simulink model "EOM_planar_vehicle"  (R2025b)
settings: Solver=VariableStepAuto  StartTime=0.0  StopTime=t_final  MaxStep=deltaTMax  RelTol=1e-3
undefined symbols (not defined in the file or in its folder): ENVIRONMENT, GEOMETRY, PROPULSION, SIMULATION
settings Model: Creator=nuris  LastModifiedBy=nuris
settings DataIOCC: ReturnWorkspaceOutputs=off

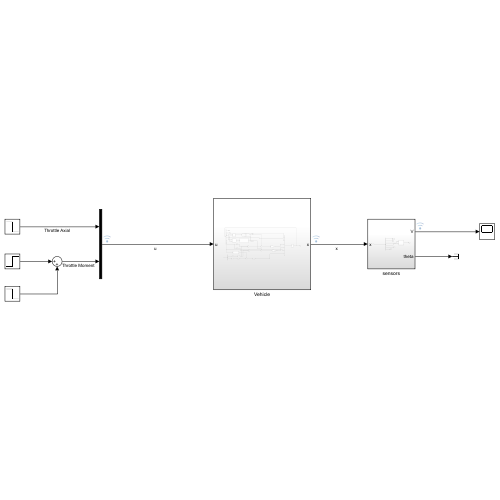
[thumbnail: Simulink's stored preview of the top-level diagram]
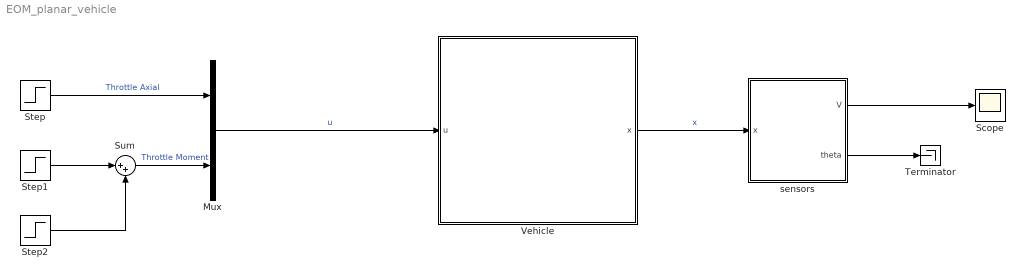
== system EOM_planar_vehicle ==
  Mux : Mux  Inputs=2
  Scope : Scope
      settings: ActiveDisplayYMinimum=-1.0187214318443125  ActiveDisplayYMaximum=20.5772184986616
  Step : Step  Time=90  Before=1  After=0  SampleTime=0
  Step1 : Step  Time=10  SampleTime=0
  Step2 : Step  Time=30  After=-1  SampleTime=0
  Sum : Sum  Inputs=|++
  Terminator : Terminator
  Vehicle : Subsystem
  sensors : Subsystem
  wires:
  Step2/1 -> Sum/2
  Step1/1 -> Sum/1
  Sum/1 -> Mux/2  "Throttle Moment"
  Step/1 -> Mux/1  "Throttle Axial"
  Mux/1 -> Vehicle/1(u)  "u"
  Vehicle/1(x) -> sensors/1(x)  "x"
  sensors/2(theta) -> Terminator/1
  sensors/1(V) -> Scope/1

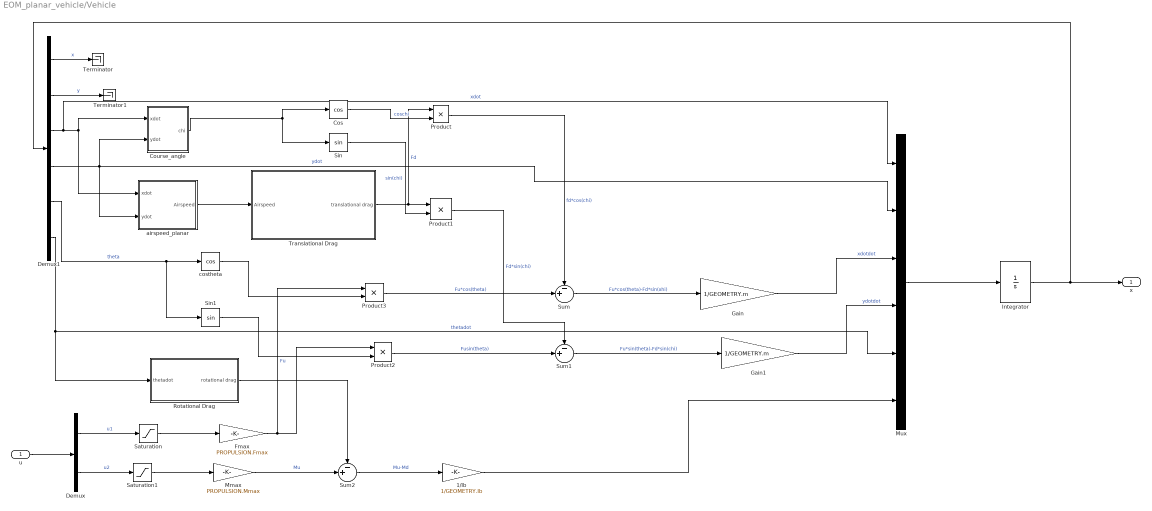
== system EOM_planar_vehicle/Vehicle ==
  u : Inport
  1/Ib : Gain  Gain=1/GEOMETRY.Ib
  Cos : Trigonometry  Operator=cos
  Course_angle : Subsystem
  Demux : Demux  Outputs=2
  Demux1 : Demux  Outputs=6
  Fmax : Gain  Gain=PROPULSION.Fmax
  Gain : Gain  Gain=1/GEOMETRY.m
  Gain1 : Gain  Gain=1/GEOMETRY.m
  Integrator : Integrator  InitialCondition=SIMULATION.X_0
  Mmax : Gain  Gain=PROPULSION.Mmax
  Mux : Mux  Inputs=6
  Product{,1..3} (4 alike) : Product
  Rotational Drag : Subsystem
  Saturation : Saturate  UpperLimit=1  LowerLimit=-1
  Saturation1 : Saturate  UpperLimit=1  LowerLimit=-1
  Sin : Trigonometry
  Sin1 : Trigonometry
  Sum : Sum  Inputs=-+|
  Sum1 : Sum  Inputs=-+|
  Sum2 : Sum  Inputs=-+|
  Terminator : Terminator
  Terminator1 : Terminator
  Translational Drag : Subsystem
  airspeed_planar : Subsystem
  costheta : Trigonometry  Operator=cos
  x : Outport
  wires:
  u/1 -> Demux/1
  Demux/1 -> Saturation/1  "u1"
  Demux/2 -> Saturation1/1  "u2"
  Saturation/1 -> Fmax/1
  Saturation1/1 -> Mmax/1
  Fmax/1 -> Product3/1, Product2/1  "Fu"
  Mmax/1 -> Sum2/2  "Mu"
  Demux1/1 -> Terminator/1  "x"
  Demux1/3 -> Mux/1, airspeed_planar/1(xdot), Course_angle/1(xdot)  "xdot"
  Demux1/4 -> airspeed_planar/2(ydot), Course_angle/2(ydot), Mux/2  "ydot"
  airspeed_planar/1(Airspeed) -> Translational Drag/1(Airspeed)
  Demux1/6 -> Mux/5, Rotational Drag/1(thetadot)  "thetadot"
  Demux1/2 -> Terminator1/1  "y"
  Course_angle/1(chi) -> Sin/1, Cos/1
  Product/1 -> Sum/1  "fd*cos(chi)"
  Translational Drag/1(translational drag) -> Product1/1, Product/1  "Fd"
  Cos/1 -> Product/2  "coschi"
  Sin/1 -> Product1/2  "sin(chi)"
  Product1/1 -> Sum1/1  "Fd*sin(chi)"
  Demux1/5 -> Sin1/1, costheta/1  "theta"
  Sin1/1 -> Product2/2
  Product2/1 -> Sum1/2  "Fusin(theta)"
  costheta/1 -> Product3/2
  Product3/1 -> Sum/2  "Fu*cos(theta)"
  Sum/1 -> Gain/1  "Fu*cos(theta)-Fd*sin(xhi)"
  Sum1/1 -> Gain1/1  "Fu*sin(theta)-Fd*sin(chi)"
  Gain/1 -> Mux/3  "xdotdot"
  Gain1/1 -> Mux/4  "ydotdot"
  Mux/1 -> Integrator/1
  Rotational Drag/1(rotational drag) -> Sum2/1
  Sum2/1 -> 1/Ib/1  "Mu-Md"
  1/Ib/1 -> Mux/6
  Integrator/1 -> Demux1/1, x/1

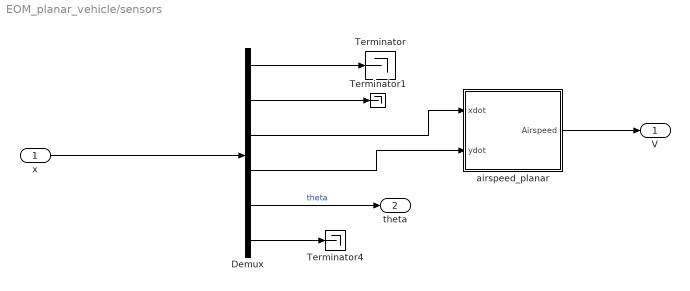
== system EOM_planar_vehicle/sensors ==
  x : Inport
  Demux : Demux  Outputs=6
  Terminator : Terminator
  Terminator1 : Terminator
  Terminator4 : Terminator
  airspeed_planar : Subsystem
  V : Outport
  theta : Outport  Port=2
  wires:
  x/1 -> Demux/1
  Demux/1 -> Terminator/1
  Demux/2 -> Terminator1/1
  Demux/3 -> airspeed_planar/1(xdot)
  Demux/4 -> airspeed_planar/2(ydot)
  Demux/5 -> theta/1  "theta"
  airspeed_planar/1(Airspeed) -> V/1
  Demux/6 -> Terminator4/1

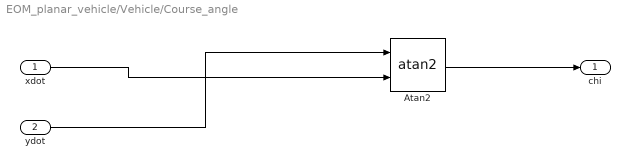
== system EOM_planar_vehicle/Vehicle/Course_angle ==
  xdot : Inport
  ydot : Inport  Port=2
  Atan2 : Trigonometry  Operator=atan2
  chi : Outport
  wires:
  ydot/1 -> Atan2/1
  Atan2/1 -> chi/1
  xdot/1 -> Atan2/2

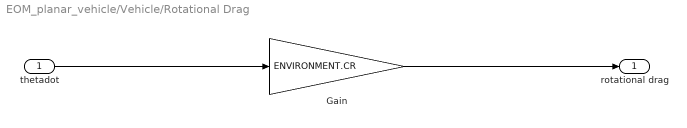
== system EOM_planar_vehicle/Vehicle/Rotational Drag ==
  thetadot : Inport
  Gain : Gain  Gain=ENVIRONMENT.CR
  rotational drag : Outport
  wires:
  Gain/1 -> rotational drag/1
  thetadot/1 -> Gain/1

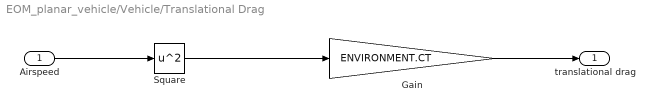
== system EOM_planar_vehicle/Vehicle/Translational Drag ==
  Airspeed : Inport
  Gain : Gain  Gain=ENVIRONMENT.CT
  Square : Math  Operator=square
  translational drag : Outport
  wires:
  Airspeed/1 -> Square/1
  Square/1 -> Gain/1
  Gain/1 -> translational drag/1

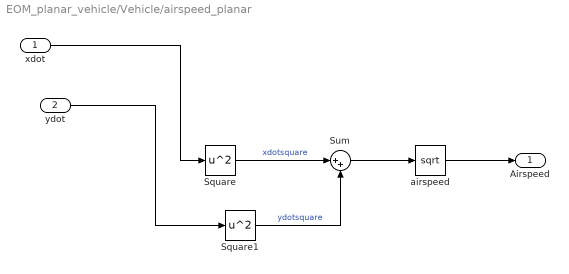
== system EOM_planar_vehicle/Vehicle/airspeed_planar ==
  xdot : Inport
  ydot : Inport  Port=2
  Square : Math  Operator=square
  Square1 : Math  Operator=square
  Sum : Sum  Inputs=|++
  airspeed : Sqrt
  Airspeed : Outport
  wires:
  ydot/1 -> Square1/1
  xdot/1 -> Square/1
  Square/1 -> Sum/1  "xdotsquare"
  Square1/1 -> Sum/2  "ydotsquare"
  Sum/1 -> airspeed/1
  airspeed/1 -> Airspeed/1

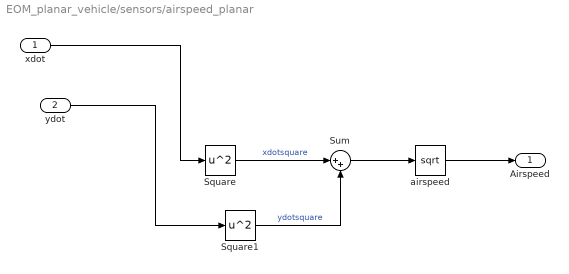
== system EOM_planar_vehicle/sensors/airspeed_planar ==
  xdot : Inport
  ydot : Inport  Port=2
  Square : Math  Operator=square
  Square1 : Math  Operator=square
  Sum : Sum  Inputs=|++
  airspeed : Sqrt
  Airspeed : Outport
  wires:
  ydot/1 -> Square1/1
  xdot/1 -> Square/1
  Square/1 -> Sum/1  "xdotsquare"
  Square1/1 -> Sum/2  "ydotsquare"
  Sum/1 -> airspeed/1
  airspeed/1 -> Airspeed/1
